simulink model "three_p_diode_rect_buck"  (R2022b)
settings: Solver=FixedStepAuto  StartTime=0.0  StopTime=0.5  RelTol=1e-3
libraries: spsDiodeLib x8, spsSeriesRLCBranchLib x6, spsVoltageMeasurementLib x5, spsACVoltageSourceLib x3, spsCurrentMeasurementLib x3, spsDCVoltageSourceLib x3, spsMosfetLib x2, spsDCMachineLib x1, sps_lib x1
settings Model: Creator=alman  LastModifiedBy=alman
settings SolverCC: ZeroCrossAlgorithm=Adaptive
settings DebuggingCC: IgnoredZcDiagnostic=none

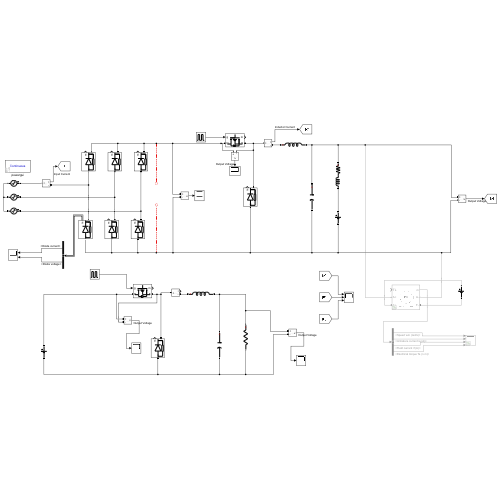
[thumbnail: Simulink's stored preview of the top-level diagram]
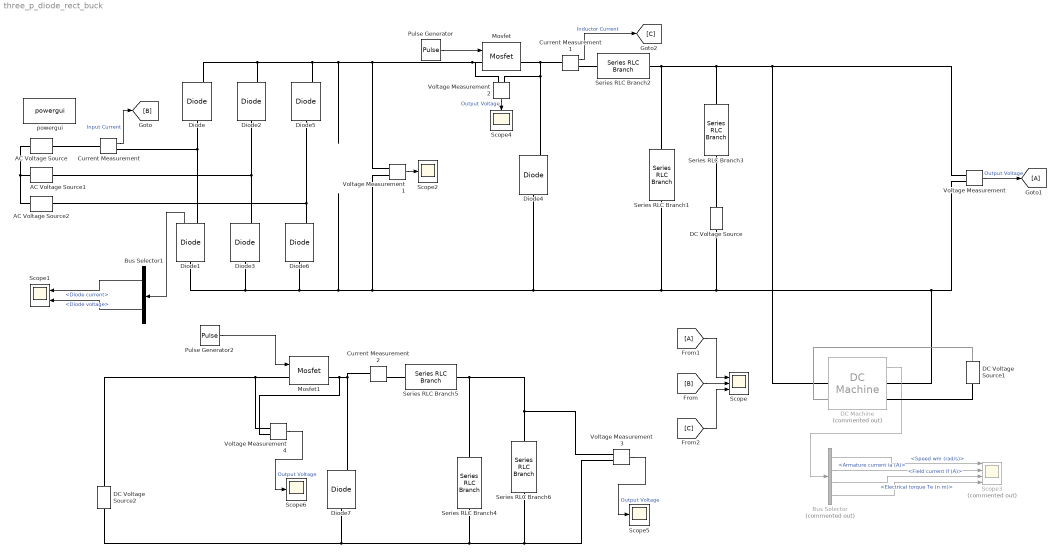
== system three_p_diode_rect_buck ==
  AC Voltage Source : spsACVoltageSourceLib/AC Voltage Source  Amplitude=230*sqrt(2)  Phase=0  Frequency=50  SampleTime=0  Measurements=None  BusType=swing  Pref=10e3  Qref=0  Qmin=-inf  Qmax=+inf
  AC Voltage Source1 : spsACVoltageSourceLib/AC Voltage Source  Amplitude=230*sqrt(2)  Phase=-120  Frequency=50  SampleTime=0  Measurements=None  BusType=swing  Pref=10e3  Qref=0  Qmin=-inf  Qmax=+inf
  AC Voltage Source2 : spsACVoltageSourceLib/AC Voltage Source  Amplitude=230*sqrt(2)  Phase=-240  Frequency=50  SampleTime=0  Measurements=None  BusType=swing  Pref=10e3  Qref=0  Qmin=-inf  Qmax=+inf
  Bus Selector : BusSelector  Commented=on  OutputSignals=Speed wm (rad/s),Armature current ia (A),Field current if (A),Electrical torque Te (n m)
  Bus Selector1 : BusSelector  OutputSignals=Diode current,Diode voltage
  Current Measurement : spsCurrentMeasurementLib/Current Measurement  PhasorSimulation=off  OutputType=Complex  PSBequivalent=0
  Current Measurement1 : spsCurrentMeasurementLib/Current Measurement  PhasorSimulation=off  OutputType=Complex  PSBequivalent=0
  Current Measurement2 : spsCurrentMeasurementLib/Current Measurement  PhasorSimulation=off  OutputType=Complex  PSBequivalent=0
  DC Machine : spsDCMachineLib/DC Machine  Commented=on  PresetModel=No  MechanicalLoad=Torque TL  FieldType=Wound  ShowDetailedParameters=on  MeasurementBus=off  RLa="[ 1.07  0.0245]"  RLf="[ 240  120]"  Laf=1.8  MachineConstant=Torque constant (N.m/A)  Ke=1.8  Kt=1.8  J=1  Bm=0  Tf=0  w0=1  Ifinit=1.66666666502173  TsPowergui=0  TsBlock=-1
  DC Voltage Source : spsDCVoltageSourceLib/DC Voltage Source  Amplitude=160  Measurements=None
  DC Voltage Source1 : spsDCVoltageSourceLib/DC Voltage Source  Amplitude=100  Measurements=None
  DC Voltage Source2 : spsDCVoltageSourceLib/DC Voltage Source  Amplitude=530  Measurements=None
  Diode{,1..7} (8 alike) : spsDiodeLib/Diode  Ron=0.001  Lon=0  Vf=0.8  IC=0  UseSnubber=0  Rs=500  Cs=250e-9  Measurements=on
  From1 : From
  Goto1 : Goto
  Mosfet : spsMosfetLib/Mosfet  Ron=0.1  Lon=0  Rd=0.01  Vfd=0  IC=0  Rs=1e5  Cs=inf  Measurements=on
  Mosfet1 : spsMosfetLib/Mosfet  Ron=0.1  Lon=0  Rd=0.01  Vfd=0  IC=0  Rs=1e5  Cs=inf  Measurements=on
  Pulse Generator : DiscretePulseGenerator  PulseType=Time based  Period=1/1000  PulseWidth=33
  Pulse Generator2 : DiscretePulseGenerator  PulseType=Time based  Period=1/10000  PulseWidth=33
  Scope : Scope  NumInputPorts=3
  Scope1 : Scope  NumInputPorts=2
  Scope{2,4..6} (4 alike) : Scope
  Scope3 : Scope  Commented=on  NumInputPorts=4
  Series RLC Branch1 : spsSeriesRLCBranchLib/Series RLC Branch  LConnTagsString=__new0  RConnTagsString=__new0  BranchType=C  Resistance=1  Inductance=1e-3  SetiL0=off  InitialCurrent=0  Capacitance=100E-6  Setx0=off  InitialVoltage=0  Measurements=None
  Series RLC Branch2 : spsSeriesRLCBranchLib/Series RLC Branch  LConnTagsString=__new0  RConnTagsString=__new0  BranchType=L  Resistance=1  Inductance=33e-3  SetiL0=off  InitialCurrent=0  Capacitance=1e-6  Setx0=off  InitialVoltage=0  Measurements=Branch current
  Series RLC Branch3 : spsSeriesRLCBranchLib/Series RLC Branch  LConnTagsString=__new0  RConnTagsString=__new0  BranchType=RL  Resistance=1.07  Inductance=24.5e-3  SetiL0=off  InitialCurrent=0  Capacitance=1e-6  Setx0=off  InitialVoltage=0  Measurements=None
  Series RLC Branch4 : spsSeriesRLCBranchLib/Series RLC Branch  LConnTagsString=__new0  RConnTagsString=__new0  BranchType=C  Resistance=1  Inductance=1e-3  SetiL0=off  InitialCurrent=0  Capacitance=100e-6  Setx0=off  InitialVoltage=0  Measurements=None
  Series RLC Branch5 : spsSeriesRLCBranchLib/Series RLC Branch  LConnTagsString=__new0  RConnTagsString=__new0  BranchType=L  Resistance=1  Inductance=10e-3  SetiL0=off  InitialCurrent=0  Capacitance=1e-6  Setx0=off  InitialVoltage=0  Measurements=None
  Series RLC Branch6 : spsSeriesRLCBranchLib/Series RLC Branch  LConnTagsString=__new0  RConnTagsString=__new0  BranchType=R  Resistance=100  Inductance=24.5e-3  SetiL0=off  InitialCurrent=0  Capacitance=1e-6  Setx0=off  InitialVoltage=0  Measurements=None
  Voltage Measurement{,1..4} (5 alike) : spsVoltageMeasurementLib/Voltage Measurement  PhasorSimulation=off  OutputType=Complex  PSBequivalent=0
  powergui : sps_lib/powergui  Priority=1  SimulationMode=Continuous  SampleTime=50e-6  frequency=60  Iterations=50  frequencyindice=0  Pbase=100e6  ErrMax=1e-4  UnitsV=kV  UnitsW=MW  buscounter=0  FunctionMessages=off  echomessages=off  EnableUseOfTLC=off  CurrentSourceSwitches=off  DisableSnubberDevices=off  DisableRonSwitches=off  DisableVfSwitches=off  DisplayEquations=off  AutomaticDiscreteSolvers=off  SolverType=Tustin/Backward Euler (TBE)  Interpol=off  ExternalGateDelay=off  methode=off  Ts=100  x0status=blocks  SPID=on  SwTol=0  HookPort=off  NonlinearTolerance=1e-4  nMaxIteration=100  ContinueOnMaxIteration=off  RestoreLinks=warning  ResistiveCurrentMeasurement=off  Frange=[0:2:500]  Ylog=off  Xlog=on  ShowGrid=off  save=off  variable=ZData  structure=0  ZoomFFT=off  StartTime=0.0  cycles=1  DisplayStyle=1  fundamental=60  FreqAxis=off  MaxFrequency=1000  frequencyindicesteady=1  RmsSteady=1  display=off
  wires:
  Voltage Measurement1/1 -> Scope2/1
  Pulse Generator/1 -> Mosfet/1
  Current Measurement1/1 -> [C]  "Inductor Current"
  Bus Selector/1 -> Scope3/1  "<Speed wm (rad/s)>"
  Bus Selector/2 -> Scope3/2  "<Armature current ia (A)>"
  Bus Selector/3 -> Scope3/3  "<Field current if (A)>"
  Bus Selector/4 -> Scope3/4  "<Electrical torque Te (n m)>"
  Voltage Measurement2/1 -> Scope4/1  "Output Voltage"
  Voltage Measurement4/1 -> Scope6/1  "Output Voltage"
  Pulse Generator2/1 -> Mosfet1/1
  Voltage Measurement3/1 -> Scope5/1  "Output Voltage"
  Current Measurement/1 -> [B]  "Input Current"
  [B] -> Scope/2
  Voltage Measurement/1 -> Goto1/1  "Output Voltage"
  From1/1 -> Scope/1
  [C] -> Scope/3
  Bus Selector1/1 -> Scope1/1  "<Diode current>"
  Bus Selector1/2 -> Scope1/2  "<Diode voltage>"
  Diode1/1 -> Bus Selector1/1
  DC Machine/1 -> Bus Selector/1
  connections:
  Diode3/RConn1 -- AC Voltage Source1/RConn1 -- Diode2/LConn1
  Diode/LConn1 -- Diode1/RConn1 -- Current Measurement/RConn1
  Mosfet/RConn1 -- Diode4/RConn1 -- Voltage Measurement2/LConn2 -- Current Measurement1/LConn1
  AC Voltage Source/LConn1 -- AC Voltage Source1/LConn1 -- AC Voltage Source2/LConn1
  AC Voltage Source/RConn1 -- Current Measurement/LConn1
  Diode6/RConn1 -- AC Voltage Source2/RConn1 -- Diode5/LConn1
  Series RLC Branch1/LConn1 -- Series RLC Branch3/LConn1 -- DC Machine/LConn1 -- Voltage Measurement/LConn1 -- Series RLC Branch2/RConn1
  Current Measurement1/RConn1 -- Series RLC Branch2/LConn1
  DC Voltage Source/RConn1 -- Series RLC Branch3/RConn1
  Diode6/LConn1 -- Voltage Measurement1/LConn2 -- Series RLC Branch1/RConn1 -- DC Machine/RConn1 -- Voltage Measurement/LConn2 -- DC Voltage Source/LConn1 -- Diode4/LConn1 -- Diode1/LConn1 -- Diode3/LConn1
  Diode5/RConn1 -- Mosfet/LConn1 -- Voltage Measurement2/LConn1 -- Voltage Measurement1/LConn1 -- Diode2/RConn1 -- Diode/RConn1
  Voltage Measurement4/LConn2 -- Mosfet1/RConn1 -- Diode7/RConn1 -- Current Measurement2/LConn1
  Series RLC Branch4/LConn1 -- Series RLC Branch5/RConn1 -- Voltage Measurement3/LConn1 -- Series RLC Branch6/LConn1
  Mosfet1/LConn1 -- DC Voltage Source2/RConn1 -- Voltage Measurement4/LConn1
  Diode7/LConn1 -- Voltage Measurement3/LConn2 -- Series RLC Branch6/RConn1 -- Series RLC Branch4/RConn1 -- DC Voltage Source2/LConn1
  Current Measurement2/RConn1 -- Series RLC Branch5/LConn1
  DC Machine/LConn2 -- DC Voltage Source1/RConn1
  DC Voltage Source1/LConn1 -- DC Machine/RConn2
